simulink model "estagio"  (R2017a)
settings: Solver=VariableStepAuto  StartTime=0.0  StopTime=24000  RelTol=1e-3
values from neighbouring files (symbols this model uses):
  beer = data.beer    [estagio_cerveja.m]
  K_loss = -Theta(1)/Ts    [estagio_cerveja.m]
undefined symbols (not defined in the file or in its folder): DiscIntNeverNeededParam, K_loss_a
libraries: dspsrcs4 x4, simulink x1
settings Model: Creator=Rafael  LastModifiedBy=Rafael

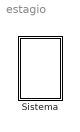
== system estagio ==
  Sistema : Subsystem

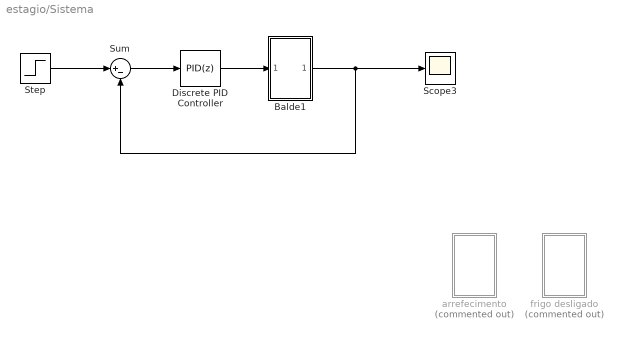
== system estagio/Sistema ==
  Balde1 : Subsystem
  Discrete PID Controller : simulink/Continuous/PID Controller  Controller=PID  TimeDomain=Discrete-time  SampleTime=-1  IntegratorMethod=Forward Euler  FilterMethod=Forward Euler  Form=Parallel  UseFilter=on  ControllerParametersSource=internal  P=30  I=0.0025  D=0  N=100  InitialConditionSource=internal  InitialConditionForIntegrator=0  InitialConditionForFilter=0  ExternalReset=none  LimitOutput=off  UpperSaturationLimit=inf  LowerSaturationLimit=-inf  LinearizeAsGain=off  AntiWindupMode=none  Kb=1  TrackingMode=off  Kt=1  PParamMin=[]  PParamMax=[]  IParamMin=[]  IParamMax=[]  DParamMin=[]  DParamMax=[]  NParamMin=[]  NParamMax=[]  KbParamMin=[]  KbParamMax=[]  KtParamMin=[]  KtParamMax=[]  POutMin=[]  POutMax=[]  IOutMin=[]  IOutMax=[]  DOutMin=[]  DOutMax=[]  NOutMin=[]  NOutMax=[]  KbOutMin=[]  KbOutMax=[]  KtOutMin=[]  KtOutMax=[]  IntegratorOutMin=[]  IntegratorOutMax=[]  FilterOutMin=[]  FilterOutMax=[]  SumOutMin=[]  SumOutMax=[]  SumI1OutMin=[]  SumI1OutMax=[]  SumI2OutMin=[]  SumI2OutMax=[]  SumI3OutMin=[]  SumI3OutMax=[]  SumDOutMin=[]  SumDOutMax=[]  SaturationOutMin=[]  SaturationOutMax=[]  IntegratorContinuousStateAttributes=''  IntegratorStateMustResolveToSignalObject=off  IntegratorRTWStateStorageClass=Auto  FilterContinuousStateAttributes=''  FilterStateMustResolveToSignalObject=off  FilterRTWStateStorageClass=Auto  DifferentiatorICPrevScaledInput=0  DifferentiatorOutMin=[]  DifferentiatorOutMax=[]  InitialConditionSetting=State (most efficient)
  Scope3 : Scope
  Step : Step  After=18  SampleTime=0
  Sum : Sum  Inputs=|+-
  arrefecimento : Subsystem  Commented=on
  frigo desligado : Subsystem  Commented=on
  wires:
  Sum/1 -> Discrete PID Controller/1
  Discrete PID Controller/1 -> Balde1/1(Tout)
  Balde1/1(Tin) -> Scope3/1, Sum/2
  Step/1 -> Sum/1

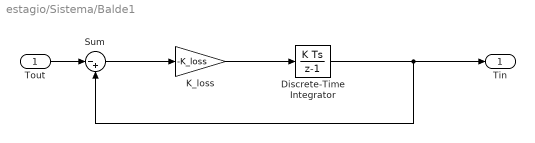
== system estagio/Sistema/Balde1 ==
  Tout : Inport
  Discrete-Time Integrator : DiscreteIntegrator  InitialCondition=25  InitialConditionSetting=State (most efficient)  ICPrevOutput=DiscIntNeverNeededParam  ICPrevScaledInput=DiscIntNeverNeededParam
  K_loss : Gain  Gain=-K_loss
  Sum : Sum  Inputs=|-+
  Tin : Outport
  wires:
  Discrete-Time Integrator/1 -> Tin/1, Sum/2
  Sum/1 -> K_loss/1
  K_loss/1 -> Discrete-Time Integrator/1
  Tout/1 -> Sum/1

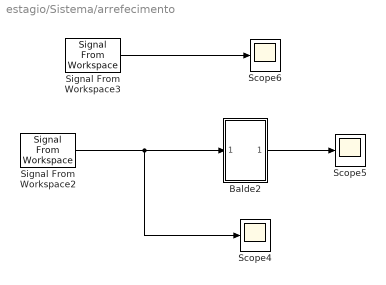
== system estagio/Sistema/arrefecimento ==
  Balde2 : Subsystem
  Scope4 : Scope
  Scope5 : Scope
  Scope6 : Scope
  Signal From Workspace2 : dspsrcs4/Signal From Workspace  X=teste_a  Ts=1  nsamps=1  OutputAfterFinalValue=Setting to zero  ignoreOrWarnInputAndFrameLengths=off  OutputFrames=off
  Signal From Workspace3 : dspsrcs4/Signal From Workspace  X=beer(1:14477)  Ts=1  nsamps=1  OutputAfterFinalValue=Setting to zero  ignoreOrWarnInputAndFrameLengths=off  OutputFrames=off
  wires:
  Balde2/1(Tin) -> Scope5/1
  Signal From Workspace2/1 -> Scope4/1, Balde2/1(Tout)
  Signal From Workspace3/1 -> Scope6/1

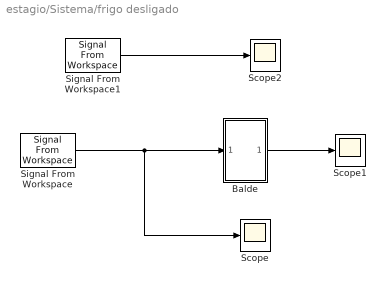
== system estagio/Sistema/frigo desligado ==
  Balde : Subsystem
  Scope : Scope
  Scope1 : Scope
  Scope2 : Scope
  Signal From Workspace : dspsrcs4/Signal From Workspace  X=teste  Ts=1  nsamps=1  OutputAfterFinalValue=Setting to zero  ignoreOrWarnInputAndFrameLengths=off  OutputFrames=off
  Signal From Workspace1 : dspsrcs4/Signal From Workspace  X=beer(14477:end)  Ts=1  nsamps=1  OutputAfterFinalValue=Setting to zero  ignoreOrWarnInputAndFrameLengths=off  OutputFrames=off
  wires:
  Signal From Workspace/1 -> Scope/1, Balde/1(Tout)
  Balde/1(Tin) -> Scope1/1
  Signal From Workspace1/1 -> Scope2/1

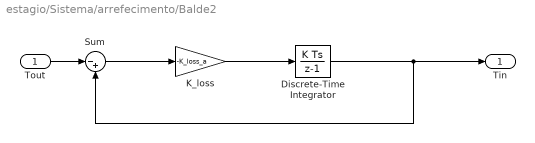
== system estagio/Sistema/arrefecimento/Balde2 ==
  Tout : Inport
  Discrete-Time Integrator : DiscreteIntegrator  InitialCondition=20.24  InitialConditionSetting=State (most efficient)  ICPrevOutput=DiscIntNeverNeededParam  ICPrevScaledInput=DiscIntNeverNeededParam
  K_loss : Gain  Gain=-K_loss_a
  Sum : Sum  Inputs=|-+
  Tin : Outport
  wires:
  Discrete-Time Integrator/1 -> Tin/1, Sum/2
  Sum/1 -> K_loss/1
  K_loss/1 -> Discrete-Time Integrator/1
  Tout/1 -> Sum/1

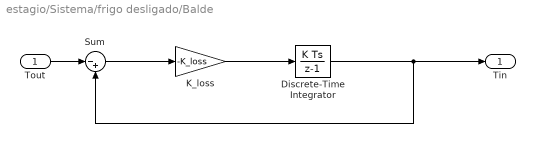
== system estagio/Sistema/frigo desligado/Balde ==
  Tout : Inport
  Discrete-Time Integrator : DiscreteIntegrator  InitialCondition=9.88  InitialConditionSetting=State (most efficient)  ICPrevOutput=DiscIntNeverNeededParam  ICPrevScaledInput=DiscIntNeverNeededParam
  K_loss : Gain  Gain=-K_loss
  Sum : Sum  Inputs=|-+
  Tin : Outport
  wires:
  Discrete-Time Integrator/1 -> Tin/1, Sum/2
  Sum/1 -> K_loss/1
  K_loss/1 -> Discrete-Time Integrator/1
  Tout/1 -> Sum/1
